simulink model "p2_4"  (R2022b)
settings: Solver=VariableStepAuto  StartTime=0.0  StopTime=10.0  RelTol=1e-3
settings Model: Creator=Ausu  LastModifiedBy=Ausu

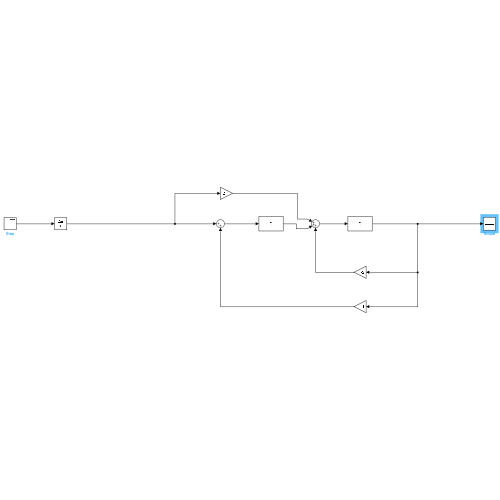
[thumbnail: Simulink's stored preview of the top-level diagram]
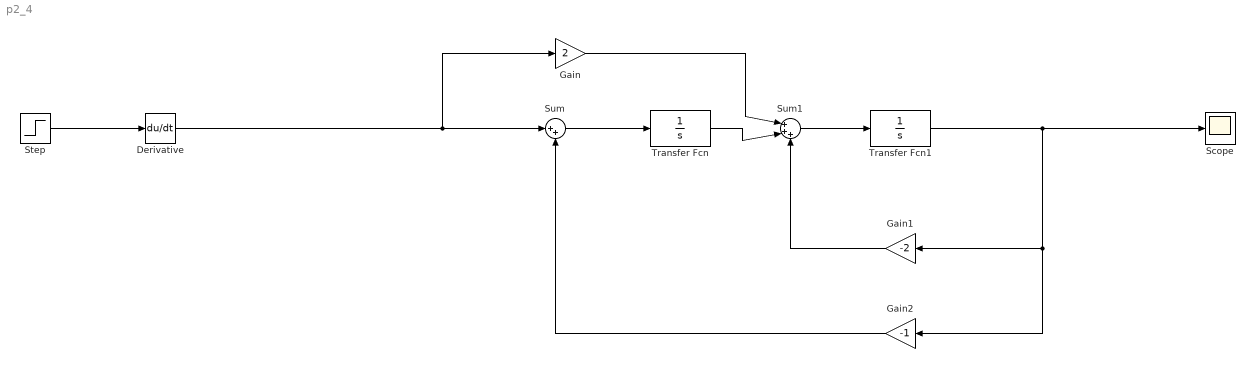
== system p2_4 ==
  Derivative : Derivative
  Gain : Gain  Gain=2
  Gain1 : Gain  Gain=-2
  Gain2 : Gain  Gain=-1
  Scope : Scope
  Step : Step  Time=0.001  SampleTime=0
  Sum : Sum  Inputs=|++
  Sum1 : Sum  Inputs=|+++
  Transfer Fcn : TransferFcn  Denominator=[1 0]
  Transfer Fcn1 : TransferFcn  Denominator=[1 0]
  wires:
  Sum1/1 -> Transfer Fcn1/1
  Gain1/1 -> Sum1/3
  Sum/1 -> Transfer Fcn/1
  Gain2/1 -> Sum/2
  Transfer Fcn/1 -> Sum1/2
  Gain/1 -> Sum1/1
  Derivative/1 -> Gain/1, Sum/1
  Step/1 -> Derivative/1
  Transfer Fcn1/1 -> Scope/1, Gain2/1, Gain1/1
